simulink model "basicmodel"  (R2018a)
settings: Solver=VariableStepAuto  StartTime=0.0  StopTime=10.0  RelTol=1e-3
settings Model: Creator=mariekutscher  LastModifiedBy=mariekutscher

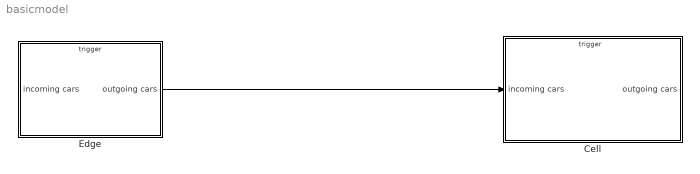
== system basicmodel ==
  Cell : Subsystem
  Edge : Subsystem
  wires:
  Edge/1(outgoing cars) -> Cell/1(incoming cars)

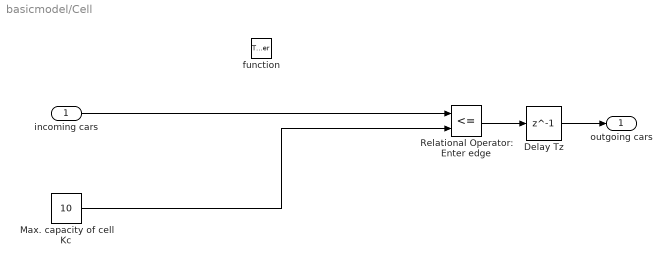
== system basicmodel/Cell ==
  incoming cars : Inport
  function : TriggerPort  TriggerType=function-call  VariantControl=Variant
  Delay Tz : Delay  DelayLength=1  InitialCondition=0
  Max. capacity of cell Kc : Constant  Value=10
  Relational Operator: Enter edge : RelationalOperator  Operator=<=  OutDataTypeStr=boolean  RndMeth=Simplest
  outgoing cars : Outport
  wires:
  Max. capacity of cell Kc/1 -> Relational Operator: Enter edge/2
  Delay Tz/1 -> outgoing cars/1
  Relational Operator: Enter edge/1 -> Delay Tz/1
  incoming cars/1 -> Relational Operator: Enter edge/1

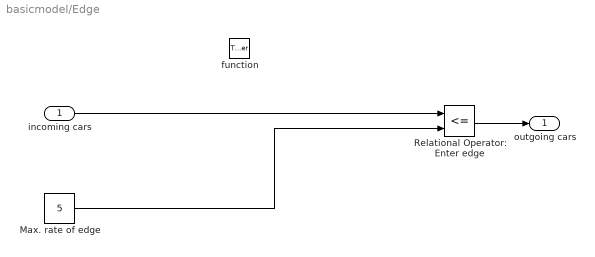
== system basicmodel/Edge ==
  "incoming cars " : Inport
  function : TriggerPort  TriggerType=function-call  VariantControl=Variant
  Max. rate of edge : Constant  Value=5
  Relational Operator: Enter edge : RelationalOperator  Operator=<=  OutDataTypeStr=boolean  RndMeth=Simplest
  outgoing cars : Outport
  wires:
  Relational Operator: Enter edge/1 -> outgoing cars/1
  Max. rate of edge/1 -> Relational Operator: Enter edge/2
  "incoming cars "/1 -> Relational Operator: Enter edge/1
